simulink model "control_scenario_1"  (R2019a)
settings: Solver=FixedStepAuto  StartTime=0.0  StopTime=10  MaxStep=0.01  RelTol=1e-4  EnableMultiTasking=on
libraries: fuzblock x1
settings Model: Creator=root  LastModifiedBy=ngiak
settings DataIOCC: LimitDataPoints=on  SaveOutput=off  SaveTime=off  ReturnWorkspaceOutputs=off
settings OptimizationCC: ExpressionDepthLimit=2147483647  LifeSpan=1
settings DebuggingCC: UnderspecifiedInitializationDetection=Classic  MergeDetectMultiDrivingBlocksExec=none  FcnCallInpInsideContextMsg=warning  AllowSymbolicDim=off  StateNameClashWarn=warning  SFUnexpectedBacktrackingDiag=warning  SFNoUnconditionalDefaultTransitionDiag=warning  SFExecutionAtInitializationDiag=none  ArithmeticOperatorsInVariantConditions=warning
settings SFSimCC: SimUseLocalCustomCode=off
settings RTWCC: RTWUseLocalCustomCode=off
settings CodeAppCC: StateflowObjectComments=on
settings GRTTargetCC: TargetLangStandard=C89/C90 (ANSI)  GeneratePreprocessorConditionals=Disable all  CombineOutputUpdateFcns=off  GRTInterface=on

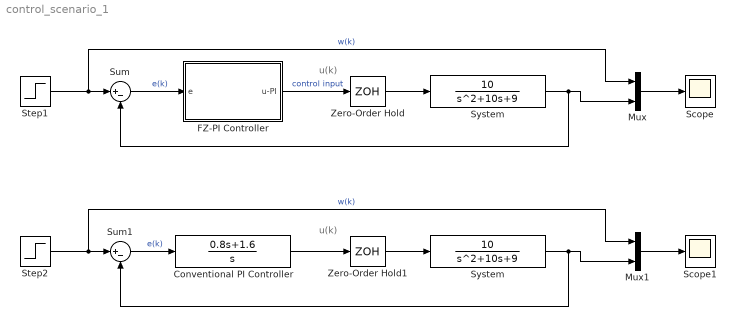
== system control_scenario_1 ==
  note: u(k)
  note: u(k)
  "Conventional PI Controller " : TransferFcn  Numerator=[0.8 1.6]  Denominator=[1 0]
  FZ-PI Controller : Subsystem
  Mux : Mux  Inputs=2
  Mux1 : Mux  Inputs=2
  Scope : Scope
  Scope1 : Scope
  Step1 : Step  Time=0  After=50  SampleTime=0
  Step2 : Step  Time=0  After=50  SampleTime=0
  Sum : Sum  Inputs=|+-
  Sum1 : Sum  Inputs=|+-
  System : TransferFcn  Numerator=[10]  Denominator=[1 10 9]
  "System " : TransferFcn  Numerator=[10]  Denominator=[1 10 9]
  Zero-Order Hold : ZeroOrderHold  SampleTime=0.01
  Zero-Order Hold1 : ZeroOrderHold  SampleTime=0.01
  wires:
  Step1/1 -> Mux/1, Sum/1  "w(k)"
  Sum/1 -> FZ-PI Controller/1(e)  "e(k)"
  FZ-PI Controller/1(u-PI) -> Zero-Order Hold/1  "control input"
  Zero-Order Hold/1 -> System/1
  System/1 -> Sum/2, Mux/2
  Mux/1 -> Scope/1
  Zero-Order Hold1/1 -> "System "/1
  Step2/1 -> Mux1/1, Sum1/1  "w(k)"
  "System "/1 -> Sum1/2, Mux1/2
  Mux1/1 -> Scope1/1
  Sum1/1 -> "Conventional PI Controller "/1  "e(k)"
  "Conventional PI Controller "/1 -> Zero-Order Hold1/1

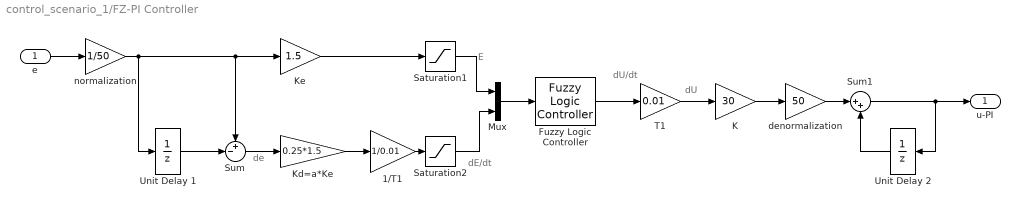
== system control_scenario_1/FZ-PI Controller ==
  note: E
  note: de
  note: dE/dt
  note: dU/dt
  note: dU
  e : Inport
  1/T1 : Gain  Gain=1/0.01
  "Fuzzy Logic Controller " : fuzblock/Fuzzy Logic  Controller  FIS='satellite.fis'  OutputSampleNumber=101  DataType=double  FuzzifiedInputs=off  RuleFiringStrengths=off  RuleOutputs=off  AggregatedOutputs=off  SimulateUsing=Interpreted execution  OutOfRangeInputValueMessage=warning  NoRuleFiredMessage=warning  EmptyOutputFuzzySetMessage=warning
  K : Gain  Gain=30
  Kd=a*Ke : Gain  Gain=0.25*1.5
  Mux : Mux  Inputs=2
  Saturation1 : Saturate  UpperLimit=1  LowerLimit=-1
  Saturation2 : Saturate  UpperLimit=1  LowerLimit=-1
  Sum : Sum  Inputs=+-|
  Sum1 : Sum  Inputs=|++
  "T1 " : Gain  Gain=0.01
  Unit Delay 1 : UnitDelay  SampleTime=0.01  HasFrameUpgradeWarning=on
  Unit Delay 2 : UnitDelay  SampleTime=0.01  HasFrameUpgradeWarning=on
  denormalization : Gain  Gain=50
  normalization : Gain  Gain=1/50
  Κe : Gain  Gain=1.5
  u-PI : Outport
  wires:
  e/1 -> normalization/1
  normalization/1 -> Unit Delay 1/1, Sum/1, Κe/1
  Unit Delay 1/1 -> Sum/2
  Sum/1 -> Kd=a*Ke/1
  Kd=a*Ke/1 -> 1/T1/1
  Κe/1 -> Saturation1/1
  1/T1/1 -> Saturation2/1
  Saturation1/1 -> Mux/1
  Saturation2/1 -> Mux/2
  "T1 "/1 -> K/1
  K/1 -> denormalization/1
  denormalization/1 -> Sum1/1
  Sum1/1 -> u-PI/1, Unit Delay 2/1
  Unit Delay 2/1 -> Sum1/2
  "Fuzzy Logic Controller "/1 -> "T1 "/1
  Mux/1 -> "Fuzzy Logic Controller "/1
